simulink model "pmsm_encoder"  (R2024b)
settings: Solver=FixedStepDiscrete  StartTime=0.0  StopTime=15  FixedStep=50e-6  RelTol=1e-3  EnableMultiTasking=on
PostLoadFcn:
  | mchp_pmsm_foc_encoder_dsPIC33A_data;
InitFcn:
  | mchp_pmsm_foc_encoder_dsPIC33A_data;
values from neighbouring files (symbols this model uses):
  PWM_frequency = 20e3    (= 20000)    [mchp_pmsm_foc_encoder_dsPIC33A_data.m]
  Ts_serialIn = 100e-3    (= 0.1)    [mchp_pmsm_foc_encoder_dsPIC33A_data.m]
undefined symbols (not defined in the file or in its folder): A0, A4, ADC, B0, C10, C11, C6, C7, C8, D11, D12, DiscIntNeverNeededParam, inverter, Max, MaxPer, ms, NumBits1, NumBits2, P1, P17, P20, P39, P40, P41, P43, P44, P60, P61, Pin, pmsm, PWM1_Trg1, Resol, s, target, us
libraries: simulink x28, MCHP_Blockset x22, mcbpositiondecoderlib x3, mcbcontrolslib x1
(part 1 of 4)
settings Model: ExtModeBatchMode=on  ExtModeEnableFloating=off  ExtModeTrigDuration=32  Creator=Lubin Kerhuel  LastModifiedBy=I52209
settings SolverCC: AlgebraicLoopSolver=TrustRegion
settings OptimizationCC: DefaultParameterBehavior=Inlined  DefaultUnderspecifiedDataType=single  EnhancedBackFolding=on  BooleansAsBitfields=on  PassReuseOutputArgsAs=Individual arguments  ZeroExternalMemoryAtStartup=off  ZeroInternalMemoryAtStartup=off  OptimizeBlockOrder=speed  DifferentSizesBufferReuse=on  EfficientTunableParamExpr=on
settings DebuggingCC: MultiTaskDSMMsg=none  MultiTaskCondExecSysMsg=none  MultiTaskRateTransMsg=warning  ParameterPrecisionLossMsg=none  ParameterTunabilityLossMsg=error  ArithmeticOperatorsInVariantConditions=warning
settings HardwareCC: ProdBitPerPointer=32  ProdBitPerSizeT=32  ProdBitPerPtrDiffT=32  ProdLargestAtomicInteger=Long  ProdWordSize=32  ProdHWDeviceType=Generic->Custom
settings ModelReferenceCC: ModelReferenceNumInstancesAllowed=Single
settings SFSimCC: MATLABDynamicMemAlloc=off  CustomCodeUndefinedFunction=UseInterfaceOnly
settings RTWCC: Description=Microchip Embedded Target dsPIC33A (real-time)  SystemTargetFile=MCHP_dsPIC33A_stf.tlc  TLCOptions="-aExtModeXCPClassicInterface=0  -aCreateExtModeTypes=1 -aExtModeXCPSimulationTimeInTicks=1"  TemplateMakefile=MCHP_dsPIC33A.tmf  DataTypeReplacement=CDataTypesFixedWidth  GPUComputeCapability=3.5
settings CodeAppCC: ForceParamTrailComments=on  IgnoreCustomStorageClasses=off  MaxIdLength=255  OperatorAnnotations=on  SimulinkDataObjDesc=on  SFDataObjDesc=on  InsertBlockDesc=on
settings STFCustomTargetCC: TargetLibSuffix=_lib.a  TargetLangStandard=C99 (ISO)  MultiwordLength=256  CombineOutputUpdateFcns=on  CombineSignalStateStructs=on  SuppressErrorStatus=on  ERTCustomFileBanners=on  SupportContinuousTime=off  RemoveResetFunc=on  MATLABClassNameForMDSCustomization=Simulink.SoftwareTarget.ERTCustomization  SystemTargetFile=MCHP_dsPIC33A_stf.tlc
settings ERTTargetCC: TargetLibSuffix=_lib.a  TargetLangStandard=C99 (ISO)  ParMdlRefBuildCompliant=off  CompOptLevelCompliant=off  ConcurrentExecutionCompliant=off  CombineSignalStateStructs=on  SuppressErrorStatus=on  SupportNonInlinedSFcns=on  ModelStepFunctionPrototypeControlCompliant=off  CPPClassGenCompliant=off  UseToolchainInfoCompliant=off  ExtModeTransport=1  ExtModeStaticAlloc=on  ExtModeStaticAllocSize=1024  ExtModeMexFile=ext_xcp  ExtModeMexArgs=1 9 2000000 './pmsm_encoder.X/pmsm_encoder.elf'  ExtModeIntrfLevel=Level2 - Open  InlinedParameterPlacement=Hierarchical  ERTSrcFileBannerTemplate=MCHP_dsPIC_code_template.cgt  ERTHdrFileBannerTemplate=MCHP_dsPIC_code_template.cgt  ERTDataSrcFileTemplate=MCHP_dsPIC_code_template.cgt  ERTDataHdrFileTemplate=MCHP_dsPIC_code_template.cgt  ERTCustomFileTemplate=MCHP_main.tlc  MaxLineWidth=110  MaxIdInt64=INT64_MAX  MinIdInt64=INT64_MIN  MaxIdUint64=UINT64_MAX  MaxIdInt32=INT32_MAX  MinIdInt32=INT32_MIN  MaxIdUint32=UINT32_MAX  MaxIdInt16=INT16_MAX  MinIdInt16=INT16_MIN  MaxIdUint16=UINT16_MAX  MaxIdInt8=INT8_MAX  MinIdInt8=INT8_MIN  MaxIdUint8=UINT8_MAX  DynamicArrayContainerType=coder::array

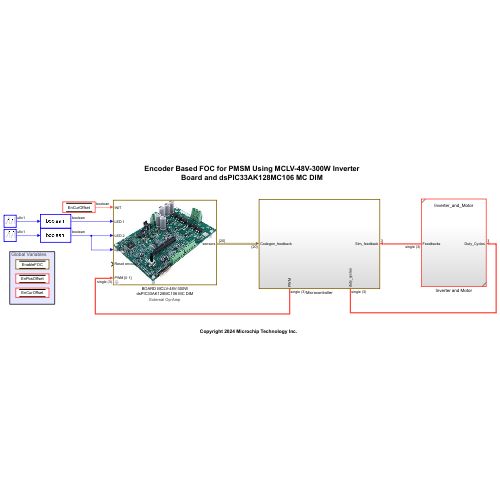
[thumbnail: Simulink's stored preview of the top-level diagram]
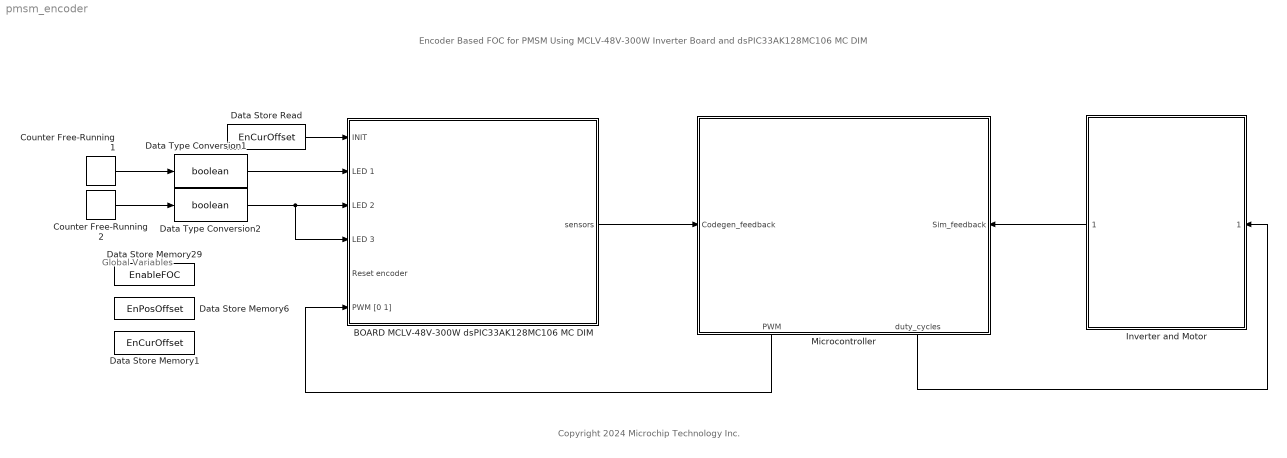
== system pmsm_encoder ==
  note: Encoder Based FOC for PMSM Using MCLV-48V-300W Inverter Board and dsPIC33AK128MC106 MC DIM
  note: Global Variables
  note: Copyright 2024 Microchip Technology Inc.
  BOARD MCLV-48V-300W dsPIC33AK128MC106 MC DIM : Subsystem  mask(MCLV-48V-300W - dsPIC33AK128MC106 MC DIM){boardVariants=External Op-Amp, n=pmsm.p, QEIResolution=pmsm.QEPSlits, Switching_Frequency=PWM_frequency, DeadTime=inverter.deadtime, QEI_Reset=on logical input (software), QEI_Offset_settings=0, QEIOffset=0}
      mask prompts: boardVariants "Board Variants"; n "Motor Pole Pairs"; QEIResolution "Optical Encoder Resolution Per Mechanical Rotation (lines)"; Switching_Frequency "PWM Switching Frequency (Hz)"; DeadTime "Dead Time (s)"; QEI_Reset "Optical encoder reset"; QEI_Offset_settings "Optical encoder offset (mechanical in rad)"; QEIOffset "Optical encoder offset (mechanical in rad)"
      mask help:
      | Template for creating Motor Control Algorithm using Microchip's MCLV-48V-300W Development Board and dsPIC33AK128MC106 Motor Control DIM.
      |
      | Template outputs:
      |   - Phase Currents (Ia and Ib)
      |   - DC Bus voltage and Bus current
      |   - Potentiometer
      |   - Push Buttons (0 when pressed, 1 for Btn 3 unconnected)
      |   - QEI Position and Velocity
      |   - MCU load and overload
      |
      | Template inputs:
      |   - INIT signal to trigger phase current offset measurement
      |   - LEDs
      |   - Reset encoder signal can be used to reset the encoder counter
      |   - PWM Duty cycle ratio [0 1]
      |
      | Note:
      | By default model and the template is configured to operate with fixed step-size of 50us.
      | This fixed step-size is synchronized with the PWM switching frequency and ADC conversion.
      |
      | Open subsystem (ctrl-u) for further customization.
      |
      | Warning:
      | Default configurations of the template are tested using the Microchip's Development Boards.
      | Any customization of the peripheral configurations needs to be verified with respect to device datasheet, hardware user guide and intended functionality.
      mask init:
      | BlksQEI = find_system(gcb,'FollowLinks','on','LookUnderMasks','all','ReferenceBlock','MCHP_Blockset/QEI/QEI');
      | QEI_Reset = get_param(gcb,'QEI_Reset');
      | if numel(BlksQEI) >= 1
      |     switch QEI_Reset
      |         case 'on index signal'
      |             set_param(BlksQEI{1},'PIMOD_mode','RESET position on each INDEX event');
      |         case 'on logical input (software)'        
      |             set_param(BlksQEI{1},'PIMOD_mode','position is cyclique between user defined boundaries'); 
      |         case 'custom setting'
      |             % do nothing 
      |     end
      | end % if
      | 
      |     BlksOpAmp = find_system(gcb,'FollowLinks','on','IncludeCommented','on','LookUnderMasks','all','ReferenceBlock','MCHP_Blockset/Analog IO/Op-Amp');
      |     if numel(BlksOpAmp) >= 1
      |         boardVariants = get_param(gcb,'boardVariants');
      |         switch boardVariants
      |             case 'internal Op-Amp'
      |                 set_param(BlksOpAmp{1},'Commented','off');
      |             case 'external Op-Amp'
      |                 set_param(BlksOpAmp{1},'Commented','on');
      |         end
      |     end % if
      settings: AttributesFormatString=%<boardVariants>
      mask Help: https://forum.microchip.com/s/sub-forums?&subForumId=a553l000000J2rNAAS&forumId=a553l000000J2pvAAC&subForumName=MATLAB&forumName=Development%20Tools&page=1&offset=0
      mask TypeOptions boardVariants: Internal Op-Amp | External Op-Amp
      mask TypeOptions QEI_Reset: on index signal | on logical input (software) | custom setting
      mask Callback QEI_Reset:
      | QEI_Reset = get_param(gcb,'QEI_Reset');
      | switch QEI_Reset
      |     case 'on index signal'
      |         QEIOffset = MCHP_Fun.Evalin('base','QEIOffset');
      |         set_param(gcb,'QEIOffset',num2str(QEIOffset));
      |         set_param(gcb,'MaskVisibilities',{'on';'on';'on';'on';'on';'on';'off';'on'});
      |     case 'on logical input (software)'
      |         set_param(gcb,'QEIOffset','0');
      |         set_param(gcb,'MaskVisibilities',{'on';'on';'on';'on';'on';'on';'off';'off'});
      |     case 'custom setting'
      |         set_param(gcb,'MaskVisibilities',{'on';'on';'on';'on';'on';'on';'off';'on'});
      |         % do nothing
      | end
      mask DialogControl boardParameters Prompt: Board
      mask DialogControl MotorParameters Prompt: Motor
      mask DialogControl n Tooltip: Number of pole pairs of the motor
      mask DialogControl QEIResolution Tooltip: encoder resolution per mechanical rotation
      mask DialogControl PWMParameters Prompt: PWM
      mask DialogControl QEIParameters Prompt: QEI
      mask DialogControl QEI_Reset Tooltip: enable encoder index signal if available. Otherwise align motor by applying a tension and set the rst input to 1
      mask DialogControl QEI_Offset_settings Tooltip: offset angle between encoder index and motor winding reference axis applied on theta_m and theta_e
      mask Display: image('MCHP_i_Board_MCLV_300W48V_reduced.jpg');
  Counter Free-Running1 : simulink/Sources/Counter Free-Running  NumBits=1  tsamp=0.5
  Counter Free-Running2 : simulink/Sources/Counter Free-Running  NumBits=1  tsamp=0.2
  Data Store Memory1 : DataStoreMemory  DataStoreName=EnCurOffset  ShowAdditionalParam=off  OutDataTypeStr=boolean
  Data Store Memory29 : DataStoreMemory  DataStoreName=EnableFOC  ShowAdditionalParam=off  OutDataTypeStr=boolean
  Data Store Memory6 : DataStoreMemory  DataStoreName=EnPosOffset  ShowAdditionalParam=off  OutDataTypeStr=boolean
  Data Store Read : DataStoreRead  DataStoreName=EnCurOffset  IndexOptions=Index vector (dialog)  Indices=1  OutputSizes=1
  Data Type Conversion1 : DataTypeConversion  OutDataTypeStr=boolean  SaturateOnIntegerOverflow=off  RndMeth=Floor
  Data Type Conversion2 : DataTypeConversion  OutDataTypeStr=boolean  SaturateOnIntegerOverflow=off  RndMeth=Floor
  Inverter and Motor : Subsystem  ReferencedSubsystem=Inverter_and_Motor
      settings: PortSchema="{\"entries\":[{\"content\":{\"sides\":[{\"content\":{\"connectorIds\":[\"Out1\"]},\"type\":\"ConnectorPlacement.EquallySpacedRectSide\",\"uuid\":\"2fd13fb8-f014-4535-a59e-aa1ad8ef2194\"},{\"content\":{\"connectorIds\":[\"In1\"],\"side\":\"RIGHT\"},\"type\":\"ConnectorPlacement.EquallySpacedRectSide\",\"uuid\":\"9b091c5a-84fb-4e1c-99c0-b531672d2343\"},{\"content\":{\"side\":\"TOP\"},\"type\":\"ConnectorPlacement.EquallySpacedRectSide\",\"uuid\":\"cbcb8365-8f8f-4340-a69e-653474eb6242\"}]},\"type\":\"ConnectorPlacement.EquallySpacedConnector\",\"uuid\":\"c1a3f948-ba30-4562-8cff-e20d0ead55ab\"}],\"packageUris\":[\"http://schema.mathworks.com/mf0/Connector/R2020b\"],\"version\":\"1.0\"}"
  Microcontroller : Subsystem
      settings: PortSchema="{\"entries\":[{\"content\":{\"sides\":[{\"content\":{\"connectorIds\":[\"In1\"]},\"type\":\"ConnectorPlacement.EquallySpacedRectSide\",\"uuid\":\"6fe6056e-88af-4075-8593-7e535d0e86a9\"},{\"content\":{\"connectorIds\":[\"In2\"],\"side\":\"RIGHT\"},\"type\":\"ConnectorPlacement.EquallySpacedRectSide\",\"uuid\":\"1f844e64-2d80-4dd2-85b1-078a1b1e54c5\"},{\"content\":{\"side\":\"TOP\"},\"type\":\"ConnectorPlacement.EquallySpacedRectSide\",\"uuid\":\"18f5eb53-6435-4f67-864b-29b16e437e19\"},{\"content\":{\"connectorIds\":[\"Out1\",\"Out2\"],\"side\":\"BOTTOM\"},\"type\":\"ConnectorPlacement.EquallySpacedRectSide\",\"uuid\":\"dce533dd-e4b2-47cf-98b1-24886c915108\"}]},\"type\":\"ConnectorPlacement.EquallySpacedConnector\",\"uuid\":\"3ecfc414-edce-4433-a88c-0c0ce6300045\"}],\"packageUris\":[\"http://schema.mathworks.com/mf0/Connector/R2020b\"],\"version\":\"1.0\"}"
  wires:
  Data Type Conversion2/1 -> BOARD MCLV-48V-300W dsPIC33AK128MC106 MC DIM/4(LED 3), BOARD MCLV-48V-300W dsPIC33AK128MC106 MC DIM/3(LED 2)
  Counter Free-Running1/1 -> Data Type Conversion1/1
  Counter Free-Running2/1 -> Data Type Conversion2/1
  Data Type Conversion1/1 -> BOARD MCLV-48V-300W dsPIC33AK128MC106 MC DIM/2(LED 1)
  BOARD MCLV-48V-300W dsPIC33AK128MC106 MC DIM/1(sensors) -> Microcontroller/1(Codegen_feedback)
  Inverter and Motor/1 -> Microcontroller/2(Sim_feedback)
  Microcontroller/2(duty_cycles) -> Inverter and Motor/1
  Microcontroller/1(PWM) -> BOARD MCLV-48V-300W dsPIC33AK128MC106 MC DIM/6(PWM [0 1])
  Data Store Read/1 -> BOARD MCLV-48V-300W dsPIC33AK128MC106 MC DIM/1(INIT)
